simulink model "lab52"  (R2018b)
settings: Solver=ode4  StartTime=0.0  StopTime=20.0  FixedStep=0.01  RelTol=1e-3
values from neighbouring files (symbols this model uses):
  A = [-4, -4, 0; 1, 0 ,0; 0, 1, 0]    [scriptlab2.m]    (also in scriptlab3.m = [-1, 0, 0; -1, -2 ,-101; 1, 1, 0]; scriptlab5.m = [0 , 0, 0; 1, 0 , -1; 0,1,2]; scriptlab7.m = [0,0,0;1,0,-1;0,1,2])
  B = [1;0;0]    [scriptlab2.m]    (also in scriptlab3.m = [0,1;1,-1;0,0]; scriptlab5.m = [0,-1;1,0;0,1]; scriptlab7.m = [0,-1;1,0;0,1])
  C = [0,1,2]    [scriptlab2.m]    (also in scriptlab3.m = [1,0,101]; scriptlab5.m = [1,0,1]; scriptlab7.m = [1,0,1])
  F = F0 + g*ft    [scriptlab5.m]    (also in scriptlab7.m)
  G = eye(m)    [scriptlab5.m]
settings Model: Creator=grecu  LastModifiedBy=grecu

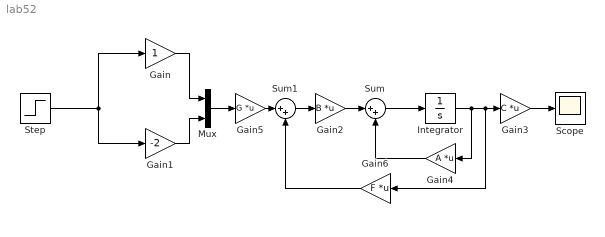
== system lab52 ==
  Gain : Gain
  Gain1 : Gain  Gain=-2
  Gain2 : Gain  Gain=B  Multiplication=Matrix(K*u)
  Gain3 : Gain  Gain=C  Multiplication=Matrix(K*u)
  Gain4 : Gain  Gain=A  Multiplication=Matrix(K*u)
  Gain5 : Gain  Gain=G  Multiplication=Matrix(K*u)
  Gain6 : Gain  Gain=F  Multiplication=Matrix(K*u)
  Integrator : Integrator
  Mux : Mux  Inputs=2
  Scope : Scope
  Step : Step  SampleTime=0
  Sum : Sum  Inputs=|++
  Sum1 : Sum  Inputs=|++
  wires:
  Gain2/1 -> Sum/1
  Integrator/1 -> Gain4/1, Gain6/1, Gain3/1
  Gain/1 -> Mux/1
  Sum/1 -> Integrator/1
  Gain3/1 -> Scope/1
  Step/1 -> Gain/1, Gain1/1
  Mux/1 -> Gain5/1
  Gain4/1 -> Sum/2
  Gain1/1 -> Mux/2
  Gain5/1 -> Sum1/1
  Sum1/1 -> Gain2/1
  Gain6/1 -> Sum1/2
